simulink model "MinSegMotor_signal_reconstruction_fractional"  (R2024a)
settings: Solver=FixedStepAuto  StartTime=0.0  StopTime=T_fin  FixedStep=T_cs  RelTol=1e-3  EnableMultiTasking=on
PostLoadFcn:
  | try,
  | codertarget.arduinobase.registry.setBaudRate(gcs,115200)
  | disp('baud rate set to 115200 for external mode hardware serial')
  | baudrate='set_to_115200'
  | catch
  | disp('baud rate setting not needed in this version')
  | end
undefined symbols (not defined in the file): B_para, f_in, L, R, T_cs, wk_fir, wk_iir
libraries: MinSegLibrary_M2V5 x2
settings Model: SimulationMode=external  ExtModeTrigDuration=2  Creator=Alec  LastModifiedBy=tpjch
settings SolverCC: AlgebraicLoopSolver=TrustRegion  AutoInsertRateTranBlk=on
settings DataIOCC: LimitDataPoints=on  SaveFormat=Array  ReturnWorkspaceOutputs=off
settings OptimizationCC: EnhancedBackFolding=on  PassReuseOutputArgsThreshold=0  ExpressionDepthLimit=2147483647  MaxStackSize=64  OptimizeBlockOrder=speed  DifferentSizesBufferReuse=on  OptimizationCustomize=off
settings DebuggingCC: UnderspecifiedInitializationDetection=Classic  MergeDetectMultiDrivingBlocksExec=none  MultiTaskRateTransMsg=warning  ParameterTunabilityLossMsg=error  UnconnectedInputMsg=warning  UnconnectedOutputMsg=warning  UnconnectedLineMsg=warning  StateNameClashWarn=warning  SFUnexpectedBacktrackingDiag=warning  SFNoUnconditionalDefaultTransitionDiag=warning  SFExecutionAtInitializationDiag=none  ArithmeticOperatorsInVariantConditions=warning
settings HardwareCC: ProdBitPerInt=16  ProdBitPerPointer=16  ProdBitPerSizeT=16  ProdBitPerPtrDiffT=16  ProdLargestAtomicFloat=None  ProdWordSize=8  ProdHWDeviceType=Atmel->AVR  UseEmbeddedCoderFeatures=off  UseSimulinkCoderFeatures=off
settings ModelReferenceCC: PropagateSignalLabelsOutOfModel=off
settings SFSimCC: SimUseLocalCustomCode=off  CustomCodeUndefinedFunction=UseInterfaceOnly
settings RTWCC: Description=Embedded Coder  SystemTargetFile=ert.tlc  HardwareBoard=Arduino Mega 2560  TemplateMakefile=ert_default_tmf  RTWVerbose=off  RTWUseLocalCustomCode=off  Toolchain=Arduino AVR  BuildConfiguration=Faster Runs  GPUComputeCapability=3.5
settings CodeAppCC: ForceParamTrailComments=on  OperatorAnnotations=on  MangleLength=10
settings ERTTargetCC: ERTCustomFileBanners=off  SupportContinuousTime=on  SupportNonInlinedSFcns=on  RemoveResetFunc=off  SupportVariableSizeSignals=on  ModelStepFunctionPrototypeControlCompliant=off  ExtMode=on  ExtModeTransport=3  ExtModeStaticAlloc=on  ExtModeAutomaticAllocSize=off  ExtModeStaticAllocSize=2048  ExtModeMexFile=ext_xcp  ExtModeMexArgs=0 6 115200  ExtModeIntrfLevel=Level2 - Open  ERTSrcFileBannerTemplate=codertarget_code_template.cgt  ERTHdrFileBannerTemplate=codertarget_code_template.cgt  ERTDataSrcFileTemplate=codertarget_code_template.cgt  ERTDataHdrFileTemplate=codertarget_code_template.cgt
settings ConfigComp: CovMetricSettings=dw  CovSaveCumulativeToWorkspaceVar=on  CovSaveSingleToWorkspaceVar=on  CovExternalEMLEnable=off

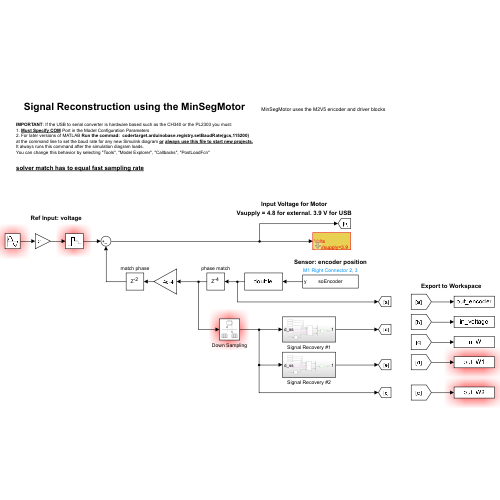
[thumbnail: Simulink's stored preview of the top-level diagram]
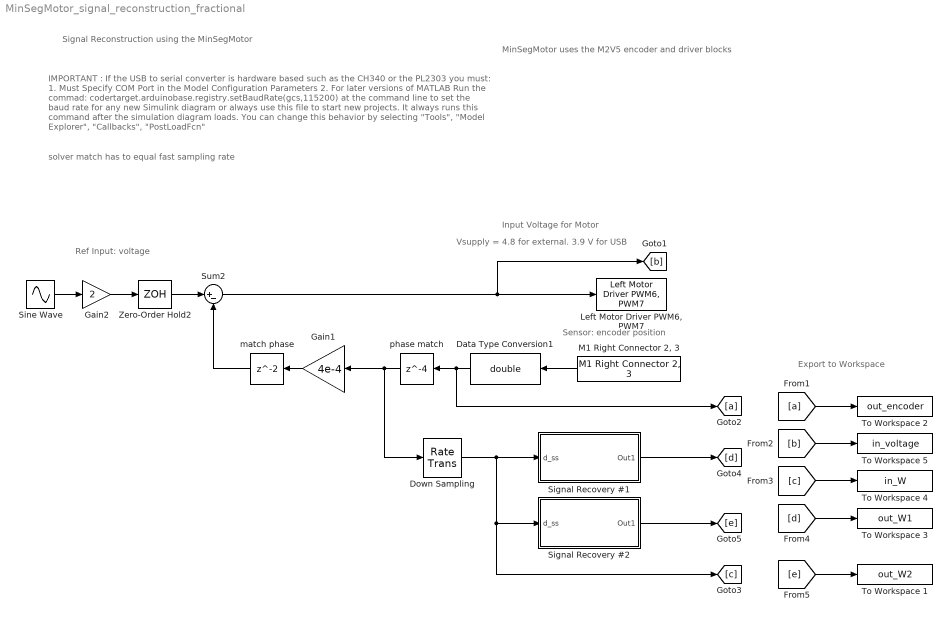
== system MinSegMotor_signal_reconstruction_fractional ==
  note: MinSegMotor uses the M2V5 encoder and driver blocks
  note: IMPORTANT : If the USB to serial converter is hardware based such as the CH340 or the PL2303 you must:
      | 1. Must Specify COM Port in the Model Configuration Parameters
      | 2. For later versions of MATLAB Run the commad: codertarget.arduinobase.registry.setBaudRate(gcs,115200)
      | at the command line to set the baud rate for any new Simulink diagram or always use this file to start new projects.
      | It always runs this command after the simulation diagram loads.
      | You can change this behavior by selecting "Tools", "Model Explorer", "Callbacks", "PostLoadFcn"
  note: solver match has to equal fast sampling rate
  note: Input Voltage for Motor
  note: Signal Reconstruction using the MinSegMotor
  note: Ref Input: voltage
  note: Vsupply = 4.8 for external. 3.9 V for USB
  note: Export to Workspace
  note: Sensor: encoder position
  Data Type Conversion1 : DataTypeConversion  OutDataTypeStr=double  RndMeth=Nearest  SaturateOnIntegerOverflow=off
  Down Sampling : RateTransition  OutPortSampleTime=T_ss
  Gain1 : Gain  Gain=4e-4
  Gain2 : Gain  Gain=2
  "Left Motor Driver PWM6, PWM7" : MinSegLibrary_M2V5/Left Motor Driver PWM6, PWM7  Vsupply=3.9  PWMoffset=0
      settings: SourceProductName=M2V5 Library
  "M1 Right Connector 2, 3" : MinSegLibrary_M2V5/M1 Right Connector 2, 3  Encoder=0  PinA=2  PinB=3
      settings: SourceProductName=M2V5 Library
  Signal Recovery #1 : Subsystem
  Signal Recovery #2 : Subsystem
  Sine Wave : Sin  Frequency=f_in*2*pi  SampleTime=0
  Sum2 : Sum  Inputs=|+-
  To Workspace 1 : ToWorkspace  VariableName=out_W2  SaveFormat=Structure With Time  SampleTime=T_cs
      settings: MaxDataPoints=Inf
  To Workspace 2 : ToWorkspace  VariableName=out_encoder  SaveFormat=Structure With Time  SampleTime=-1
      settings: MaxDataPoints=Inf
  To Workspace 3 : ToWorkspace  VariableName=out_W1  SaveFormat=Structure With Time  SampleTime=T_cs
      settings: MaxDataPoints=Inf
  To Workspace 4 : ToWorkspace  VariableName=in_W  SaveFormat=Structure With Time  SampleTime=-1
      settings: MaxDataPoints=Inf
  To Workspace 5 : ToWorkspace  VariableName=in_voltage  SaveFormat=Structure With Time  SampleTime=-1
      settings: MaxDataPoints=Inf
  Zero-Order Hold2 : ZeroOrderHold  SampleTime=T_cs
  match phase : Delay
  phase match : Delay  DelayLength=4
  wires:
  Sine Wave/1 -> Gain2/1
  Gain2/1 -> Zero-Order Hold2/1
  "M1 Right Connector 2, 3"/1 -> Data Type Conversion1/1
  Signal Recovery #1/1(Out1) -> [d]
  [a] -> To Workspace 2/1
  [b] -> To Workspace 5/1
  [c] -> To Workspace 4/1
  [d] -> To Workspace 3/1
  [e] -> To Workspace 1/1
  Gain1/1 -> match phase/1
  Data Type Conversion1/1 -> phase match/1, [a]
  Zero-Order Hold2/1 -> Sum2/1
  match phase/1 -> Sum2/2
  Sum2/1 -> [b], "Left Motor Driver PWM6, PWM7"/1
  Signal Recovery #2/1(Out1) -> [e]
  Down Sampling/1 -> Signal Recovery #1/1(d_ss), [c], Signal Recovery #2/1(d_ss)
  phase match/1 -> Gain1/1, Down Sampling/1

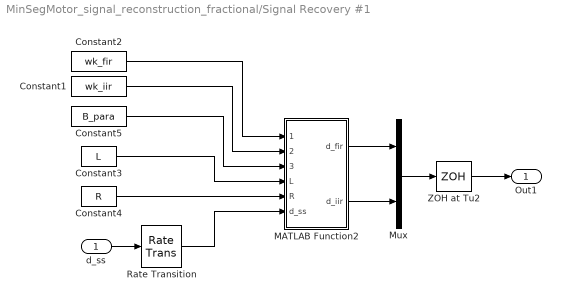
== system MinSegMotor_signal_reconstruction_fractional/Signal Recovery #1 ==
  d_ss : Inport
  Constant1 : Constant  Value=wk_iir
  Constant2 : Constant  Value=wk_fir
  Constant3 : Constant  Value=L
  Constant4 : Constant  Value=R
  Constant5 : Constant  Value=B_para
  MATLAB Function2 : MATLAB Function  TreatAsAtomicUnit=on  SystemSampleTime=T_cs
  Mux : Mux  Inputs=2
  Rate Transition : RateTransition  OutPortSampleTime=T_cs
  ZOH at Tu2 : ZeroOrderHold  SampleTime=T_cs
  Out1 : Outport
  wires:
  Constant2/1 -> MATLAB Function2/1(w_k_fir)
  ZOH at Tu2/1 -> Out1/1
  Constant3/1 -> MATLAB Function2/4(L)
  Constant4/1 -> MATLAB Function2/5(R)
  Rate Transition/1 -> MATLAB Function2/6(d_ss)
  d_ss/1 -> Rate Transition/1
  Constant1/1 -> MATLAB Function2/2(w_k_iir)
  Constant5/1 -> MATLAB Function2/3(B_para)
  MATLAB Function2/1(d_fir) -> Mux/1
  MATLAB Function2/2(d_iir) -> Mux/2
  Mux/1 -> ZOH at Tu2/1

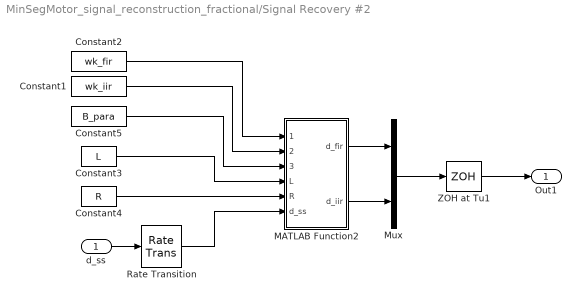
== system MinSegMotor_signal_reconstruction_fractional/Signal Recovery #2 ==
  d_ss : Inport
  Constant1 : Constant  Value=wk_iir
  Constant2 : Constant  Value=wk_fir
  Constant3 : Constant  Value=L
  Constant4 : Constant  Value=R
  Constant5 : Constant  Value=B_para
  MATLAB Function2 : MATLAB Function  TreatAsAtomicUnit=on  SystemSampleTime=T_cs
  Mux : Mux  Inputs=2
  Rate Transition : RateTransition  OutPortSampleTime=T_cs
  ZOH at Tu1 : ZeroOrderHold  SampleTime=T_cs
  Out1 : Outport
  wires:
  Constant2/1 -> MATLAB Function2/1(w_k_fir)
  Rate Transition/1 -> MATLAB Function2/6(d_ss)
  d_ss/1 -> Rate Transition/1
  Constant4/1 -> MATLAB Function2/5(R)
  Constant5/1 -> MATLAB Function2/3(B_para)
  Constant1/1 -> MATLAB Function2/2(w_k_iir)
  Constant3/1 -> MATLAB Function2/4(L)
  Mux/1 -> ZOH at Tu1/1
  MATLAB Function2/2(d_iir) -> Mux/2
  MATLAB Function2/1(d_fir) -> Mux/1
  ZOH at Tu1/1 -> Out1/1

== matlab function MinSegMotor_signal_reconstruction_fractional/Signal Recovery #1/MATLAB Function2 ==
  settings: updateMethod=DISCRETE
  data: w_k_fir input; w_k_iir input; B_para input; L input; R input; d_ss input; d_fir output size=1; d_iir output
function [d_fir, d_iir] = fcn(w_k_fir, w_k_iir, B_para, L, R, d_ss)
    % Keeps data of variables
    persistent  n_w phi n_cs n_ss d_buff d_fs_fir d_fs_iir max_buffer_size buffer_indices
    RL = R*L;
    % Assigning initial values   
    if isempty(n_w)
        n_w = size(w_k_fir,1); % n_w = 2m disturbances (index starts at 0,1,...,2m-1)
        phi = zeros(1, n_w, 'like', d_ss); % Preallocate phi using the same type as d_ss
        n_cs = 0; % combined sampling count, rate at T_fs/R
        n_ss = 0; % Slow sampling count
        d_fs_fir = 0; % store previous value for the estimate
        d_fs_iir = 0;
        buffer_indices = 2:RL:((n_w-1) * RL + 2);
        max_buffer_size = (n_w * RL + 1);
        d_buff = zeros(1, max_buffer_size, 'like', d_ss);
    end
    
    % Increment fast sampling count
    n_cs = n_cs + 1;
    k = mod(n_cs-1,2*R*L); % check if on intersample
    % Update slow sampling count when k == 0
    if k == 0
        n_ss = n_ss + 1; % Number of slow samples
    end

    % Case 1: n_ss < n_w (not enough data points for FIR)
    if n_ss < n_w
        if k == 0 % Fast and slow align
            phi = [d_ss, phi(1:end-1)]; % Shift and update phi
            d_fir = d_ss;
            d_iir = d_ss;
            d_buff = [d_iir, d_buff(1:end-1)];
        else % Not enough data for intersample estimation
            d_fir = 0;
            d_iir = 0;
            d_buff = [d_iir, d_buff(1:end-1)];
        end
    % Case 2: n_ss >= n_w (enough data points for FIR)
    elseif n_ss >= n_w && n_ss < (n_w + 1)
        if k == 0 
            phi = [d_ss, phi(1:end-1)];
            d_fir = d_ss;
            d_iir = d_ss;
            d_buff = [d_iir, d_buff(1:end-1)];
        elseif k ~= 0 && mod(k,2) == 0 % FIR reconstruction
            d_fir = phi * w_k_fir(:, k/R); 
            d_fs_fir = d_fir;
            d_iir = 0;
            d_buff = [d_iir, d_buff(1:end-1)];
        else k ~= 0 && mod(k+1,2) == 0
            d_fir = d_fs_fir;
            d_iir = 0;
        end
    % Case 3: n_w >= n_w+1, IIR reconstruction
    else
        if k == 0
            phi = [d_ss, phi(1:end-1)];
            d_fir = d_ss;
            d_iir = d_ss;
            d_buff = [d_iir, d_buff(1:end-1)];
        elseif k ~= 0 && mod(k,2) == 0
            d_fir = phi * w_k_fir(:, k/R);
            d_fs_fir = d_fir;
            d_temp = flip(d_buff);
            d_iir = phi * w_k_iir(:,k/R) - ...
                    d_temp(buffer_indices) * flip(B_para(2:end));
            d_fs_iir = d_iir;
            d_buff = [d_iir, d_buff(1:end-1)];
        else k ~= 0 && mod(k+1,2) == 0
            d_fir = d_fs_fir;
            d_iir = d_fs_iir;
        end
    end
    % update buffer
end

== matlab function MinSegMotor_signal_reconstruction_fractional/Signal Recovery #2/MATLAB Function2 ==
  settings: updateMethod=DISCRETE
  data: w_k_fir input; w_k_iir input; B_para input; L input; R input; d_ss input; d_fir output size=1; d_iir output
function [d_fir, d_iir] = fcn(w_k_fir, w_k_iir, B_para, L, R, d_ss)
    % Keeps data of variables
    persistent  n_w phi n_cs n_ss d_buff d_fs_fir d_fs_iir max_buffer_size buffer_indices
    RL = R*L; 
    % Assigning initial values   
    if isempty(n_w)
        n_w = size(w_k_fir,1); % n_w = 2m disturbances (index starts at 0,1,...,2m-1)
        phi = zeros(1, n_w, 'like', d_ss); % Preallocate phi using the same type as d_ss
        n_cs = -25; % offset to be one slow sample behind, rate at T_fs/R
        n_ss = 0; % Slow sampling count
        d_fs_fir = 0; % store previous value for the estimate
        d_fs_iir = 0;
        buffer_indices = 2:RL:((n_w-1) * RL + 2);
        max_buffer_size = (n_w * RL + 1);
        d_buff = zeros(1, max_buffer_size, 'like', d_ss);
    end
    
    % Increment fast sampling count
    n_cs = n_cs + 1;
    k = mod(n_cs-1,2*R*L); % check if on intersample
    % Update slow sampling count when k == 0
    if k == 0
        n_ss = n_ss + 1; % Number of slow samples
    end

    % Case 1: n_ss < n_w (not enough data points for FIR)
    if n_ss < n_w
        if k == 0 % Fast and slow align
            phi = [d_ss, phi(1:end-1)]; % Shift and update phi
            d_fir = d_ss;
            d_iir = d_ss;
            d_buff = [d_iir, d_buff(1:end-1)];
        else % Not enough data for intersample estimation
            d_fir = 0;
            d_iir = 0;
            d_buff = [d_iir, d_buff(1:end-1)];
        end
    % Case 2: n_ss >= n_w (enough data points for FIR)
    elseif n_ss >= n_w && n_ss < (n_w + 1)
        if k == 0 
            phi = [d_ss, phi(1:end-1)];
            d_fir = d_ss;
            d_iir = d_ss;
            d_buff = [d_iir, d_buff(1:end-1)];
        elseif k ~= 0 && mod(k,2) == 0 % FIR reconstruction
            d_fir = phi * w_k_fir(:, k/R); 
            d_fs_fir = d_fir;
            d_iir = 0;
            d_buff = [d_iir, d_buff(1:end-1)];
        else k ~= 0 && mod(k+1,2) == 0
            d_fir = d_fs_fir;
            d_iir = 0;
        end
    % Case 3: n_w >= n_w+1, IIR reconstruction
    else
        if k == 0
            phi = [d_ss, phi(1:end-1)];
            d_fir = d_ss;
            d_iir = d_ss;
            d_buff = [d_iir, d_buff(1:end-1)];
        elseif k ~= 0 && mod(k,2) == 0
            d_fir = phi * w_k_fir(:, k/R);
            d_fs_fir = d_fir;
            d_temp = flip(d_buff);
            d_iir = phi * w_k_iir(:,k/R) - ...
                    d_temp(buffer_indices) * flip(B_para(2:end));
            d_fs_iir = d_iir;
            d_buff = [d_iir, d_buff(1:end-1)];
        else k ~= 0 && mod(k+1,2) == 0
            d_fir = d_fs_fir;
            d_iir = d_fs_iir;
        end
    end
end
